simulink model "Inverted_pendulum"  (R2019b)
settings: Solver=VariableStepAuto  StartTime=0.0  StopTime=inf  RelTol=1e-3
values from neighbouring files (symbols this model uses):
  m = 100    [harmonic.m]
undefined symbols (not defined in the file or in its folder): g, K, l, Mcart, Ts
settings Model: Creator=apple  LastModifiedBy=apple

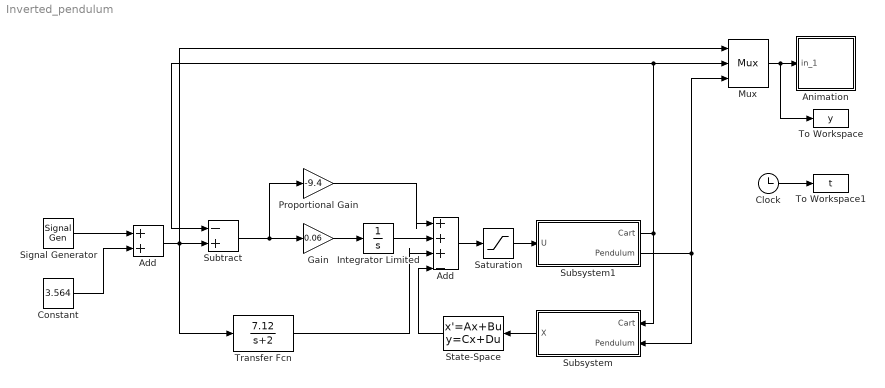
== system Inverted_pendulum ==
  Add : Sum  Inputs=+++-
  "Add " : Sum
  Animation : Subsystem  mask(Pendulum plot){RefBlock=Reference}
      mask prompts: RefBlock "DC reference signal block name:"
      mask help: Pendulum plot
      mask Help: Pendulum animation function using Handle graphics.
      mask Display: plot([-10 10],[0 0],[-2 -2 2 2],[0 1 1 0],[0 3],[1 5])
  Clock : Clock
  Constant : Constant  Value=3.564
  Gain : Gain  Gain=0.06  OutDataTypeStr=Inherit: Same as input  ParamDataTypeStr=Inherit: Same as input
  Integrator Limited : Integrator  LimitOutput=on  UpperSaturationLimit=5  LowerSaturationLimit=-5
  Mux : Mux  Inputs=3
  Proportional Gain : Gain  Gain=-9.4  OutDataTypeStr=Inherit: Same as input  ParamDataTypeStr=Inherit: Same as input
  Saturation : Saturate  UpperLimit=10  LowerLimit=-10
  "Signal Generator " : SignalGenerator  Amplitude=0.00000  Frequency=0.40000  Units=rad/sec
  State-Space : StateSpace  A=[]  B=[]  C=[]  D=K  InitialCondition=0
  Subsystem : Subsystem
  Subsystem1 : Subsystem
  Subtract : Sum  Inputs=-+
  To Workspace : ToWorkspace  VariableName=y  SampleTime=0.1
  To Workspace1 : ToWorkspace  VariableName=t  SampleTime=0.1
  Transfer Fcn : TransferFcn  Numerator=[7.12]  Denominator=[1 2]  ContinuousStateAttributes="\""
  wires:
  Constant/1 -> "Add "/2
  "Add "/1 -> Mux/1, Transfer Fcn/1, Subtract/2
  Subtract/1 -> Proportional Gain/1, Gain/1
  Gain/1 -> Integrator Limited/1
  "Signal Generator "/1 -> "Add "/1
  Saturation/1 -> Subsystem1/1(U)
  Integrator Limited/1 -> Add/2
  Proportional Gain/1 -> Add/1
  Transfer Fcn/1 -> Add/3
  Subsystem/1(X) -> State-Space/1
  State-Space/1 -> Add/4
  Add/1 -> Saturation/1
  Subsystem1/1(Cart) -> Subsystem/1(Cart), Mux/2, Subtract/1
  Subsystem1/2(Pendulum) -> Subsystem/2(Pendulum), Mux/3
  Mux/1 -> To Workspace/1, Animation/1(in_1)
  Clock/1 -> To Workspace1/1

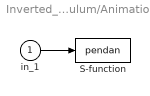
== system Inverted_pendulum/Animation ==
  in_1 : Inport
  S-function : S-Function  FunctionName=pendan  Parameters=RefBlock  SFunctionDeploymentMode=off  EnableBusSupport=off
      settings: DeleteFcn=pendan([],[],[],'DeleteBlock');
  wires:
  in_1/1 -> S-function/1

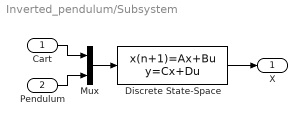
== system Inverted_pendulum/Subsystem ==
  Cart : Inport
  Pendulum : Inport  Port=2
  "Discrete State-Space " : DiscreteStateSpace  A=zeros(2)  B=-eye(2)/Ts  C=[0 0; 1 0; 0 0; 0 1]  D=[1 0; 1/Ts 0; 0 1; 0 1/Ts]  SampleTime=Ts
  Mux : Mux  Inputs=2
  X : Outport
  wires:
  Cart/1 -> Mux/1
  Pendulum/1 -> Mux/2
  Mux/1 -> "Discrete State-Space "/1
  "Discrete State-Space "/1 -> X/1

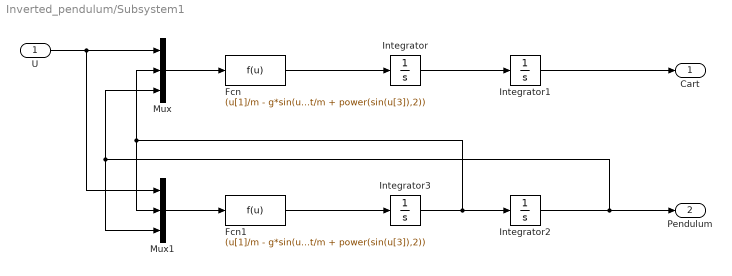
== system Inverted_pendulum/Subsystem1 ==
  U : Inport
  Fcn : Fcn  Expr=(u[1]/m - g*sin(u[3])*cos(u[3]) + l*power(u[2],2)*sin(u[3]))/(Mcart/m + power(sin(u[3]),2))
  Fcn1 : Fcn  Expr=(u[1]/m - g*sin(u[3])*cos(u[3]) + l*power(u[2],2)*sin(u[3]))/(Mcart/m + power(sin(u[3]),2))
  Integrator{,1..3} (4 alike) : Integrator
  Mux : Mux  Inputs=3
  Mux1 : Mux  Inputs=3
  Cart : Outport
  Pendulum : Outport  Port=2
  wires:
  U/1 -> Mux1/1, Mux/1
  Mux/1 -> Fcn/1
  Fcn/1 -> Integrator/1
  Integrator/1 -> Integrator1/1
  Integrator1/1 -> Cart/1
  Integrator2/1 -> Mux1/3, Mux/3, Pendulum/1
  Integrator3/1 -> Mux1/2, Mux/2, Integrator2/1
  Fcn1/1 -> Integrator3/1
  Mux1/1 -> Fcn1/1
